simulink model "power_VariableInductor"  (Simulink 6.0)
settings: Solver=ode45  SolverMode=SingleTasking  StartTime=0.0  StopTime=2  RelTol=1e-3  AbsTol=1e-6
libraries: powerlib x14
settings Model: Creator=patrice  LastModifiedBy=batserve  ExtModeTrigMode=oneshot  ExtModeArmWhenConnect=off  ExtModeAutoUpdateStatusClock=off
settings DataIOCC: LimitDataPoints=off  SignalLoggingName=sigsOut
settings OptimizationCC: BlockReduction=off  BooleanDataType=off
settings DebuggingCC: CheckExecutionContextPreStartOutputMsg=on  CheckExecutionContextRuntimeOutputMsg=on  SolverPrmCheckMsg=none
settings HardwareCC: TargetUnknown=on
settings ModelReferenceCC: UpdateModelReferenceTargets=IfOutOfDate
settings RTWCC: TemplateMakefile=grt_unix.tmf

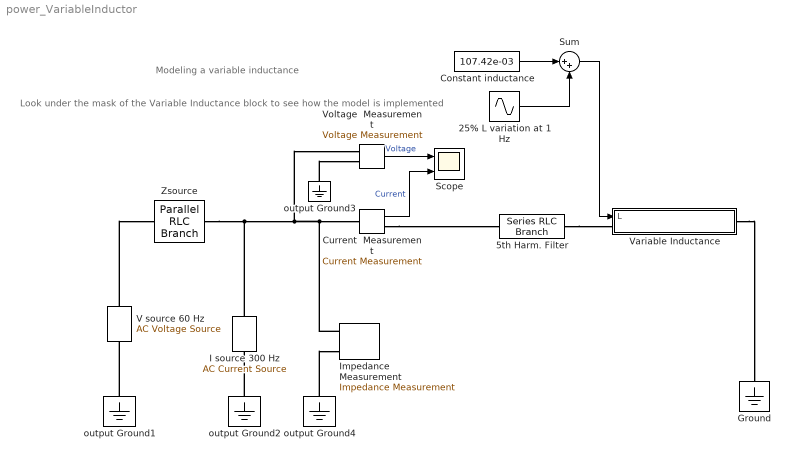
== system power_VariableInductor ==
  note: Modeling a variable inductance
  note: Look under the mask of  the Variable
      | Inductance block to see
      |  how the model is implemented
  25% L variation at 1 Hz : Sin  Amplitude=107.42e-03 *25/100  Frequency=2*pi*1  SampleTime=0
  5th Harm. Filter : powerlib/Elements/Series RLC Branch  PhysicalDomain=powersysdomain  SubClassName=unknown  LeftPortType=p1  RightPortType=p1  LConnTagsString=__new0  RConnTagsString=__new0  Resistance=1.27  Inductance=0  Capacitance=2.62e-6  Measurements=None
  "Constant inductance " : Constant  Value=107.42e-03
  Current  Measurement : powerlib/Measurements/Current Measurement  PhasorSimulation=off  OutputType=Magnitude  PSBequivalent=0
  Ground : powerlib/Elements/Ground  Orientation=down  PhysicalDomain=powersysdomain  SubClassName=unknown  LeftPortType=p1  RightPortType=p1  LConnTagsString=a
  I source 300 Hz : powerlib/Electrical Sources/AC Current Source  Orientation=up  Amplitude=10  Phase=-30  Frequency=300  SampleTime=0  Measurements=None
  Impedance  Measurement : powerlib/Measurements/Impedance Measurement  PhysicalDomain=powersysdomain  SubClassName=unknown  LeftPortType=p1  RightPortType=p1  LConnTagsString=+|-  Factor=1
  Scope : Scope  NumInputPorts=2
      settings: TimeRange=2  YMin=-500~-20  YMax=500~20  DataFormat=Array
  Sum : Sum  Inputs=|++  SaturateOnIntegerOverflow=on
  V source 60 Hz : powerlib/Electrical Sources/AC Voltage Source  Orientation=up  Amplitude=100  Phase=0  Frequency=60  SampleTime=0  Measurements=None
  Variable Inductance : Subsystem  mask{Iinit=-4.169}
      mask prompts: Iinit "Initial Voltage"
      mask Display: disp('Variable Inductor')
  Voltage  Measurement : powerlib/Measurements/Voltage Measurement  PhasorSimulation=off  OutputType=Magnitude  PSBequivalent=0
  Zsource : powerlib/Elements/Parallel RLC Branch  PhysicalDomain=powersysdomain  SubClassName=unknown  LeftPortType=p1  RightPortType=p1  LConnTagsString=a  RConnTagsString=__new0  Resistance=37.7  Inductance=10e-03  Capacitance=0  Measurements=None
  output Ground{1..4} (4 alike) : powerlib/Elements/Ground  Orientation=down  PhysicalDomain=powersysdomain  SubClassName=unknown  LeftPortType=p1  RightPortType=p1  LConnTagsString=a
  wires:
  "Constant inductance "/1 -> Sum/1
  Sum/1 -> Variable Inductance/1(L)
  25% L variation at 1 Hz/1 -> Sum/2
  Voltage  Measurement/1 -> Scope/1  "Voltage"
  Current  Measurement/1 -> Scope/2  "Current"
  connections:
  V source 60 Hz/RConn1 -- Zsource/LConn1
  Zsource/RConn1 -- Impedance  Measurement/LConn1 -- Current  Measurement/LConn1 -- Voltage  Measurement/LConn1 -- I source 300 Hz/RConn1
  output Ground1/LConn1 -- V source 60 Hz/LConn1
  output Ground2/LConn1 -- I source 300 Hz/LConn1
  output Ground3/LConn1 -- Voltage  Measurement/LConn2
  Current  Measurement/RConn1 -- 5th Harm. Filter/LConn1
  output Ground4/LConn1 -- Impedance  Measurement/LConn2
  Variable Inductance/RConn1 -- Ground/LConn1
  5th Harm. Filter/RConn1 -- Variable Inductance/LConn1

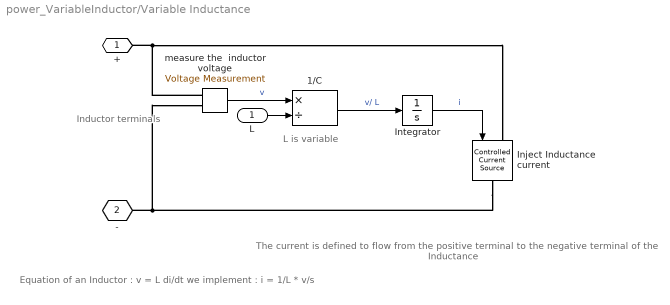
== system power_VariableInductor/Variable Inductance ==
  note: Equation of an Inductor :
      |
      | v = L di/dt
      |
      | we implement :
      |
      | i = 1/L * v/s
  note: L is variable
  note: Inductor
      | terminals
  note: The current is defined to flow from
      |  the positive terminal to the negative
      | terminal of the Inductance
  L : Inport  Port=1  LatchInput=off
  1/C : Product  Inputs=*/  SaturateOnIntegerOverflow=on
  "Inject Inductance current " : powerlib/Electrical Sources/Controlled Current Source  Orientation=down  Initialize=on  Amplitude=0  Phase=0  Frequency=0  Measurements=None
  Integrator : Integrator  InitialCondition=Iinit
  measure the  inductor voltage : powerlib/Measurements/Voltage Measurement  PhasorSimulation=off  OutputType=Magnitude  PSBequivalent=0
  + : PMIOPort  Port=1  Side=Left
  - : PMIOPort  Port=2  Side=Right
  wires:
  1/C/1 -> Integrator/1  "v/ L"
  L/1 -> 1/C/2
  measure the  inductor voltage/1 -> 1/C/1  "v"
  Integrator/1 -> "Inject Inductance current "/1  "i"
  connections:
  measure the  inductor voltage/LConn1 -- +/RConn1 -- "Inject Inductance current "/LConn1
  "Inject Inductance current "/RConn1 -- -/RConn1 -- measure the  inductor voltage/LConn2
